simulink model "Encoder_X4"  (R2025a)
settings: Solver=FixedStepAuto  StartTime=0.0  StopTime=inf  FixedStep=0.001  RelTol=1e-3  EnableMultiTasking=on
libraries: stm32f4xxblockslib x5, stm32g4xxblockslib x2, simulink x1
settings Model: STM32="{\"EncoderBlockForG4\":[{\"ID\":\"untitled:1\"},{\"ID\":\"Lab3_Encoder:1\"},{\"ID\":\"Encoder:1\"},{\"ID\":\"Encoder_1:1\"},{\"ID\":\"Encoder_X4:147\"},{\"ID\":\"Encoder_X4:1\"},{\"ID\":\"Encoder_X1:147\"},{\"ID\":\"Encoder_X1:1\"},{\"ID\":\"Encoder_X2:147\"},{\"ID\":\"Encoder_X2:1\"}],\"DigitalPortRead\":[{\"ID\":\"Encoder:46\"},{\"ID\":\"Encoder:50\"},{\"ID\":\"Encoder:56\"},{\"ID\":\"Encoder_1:56\"},{\"ID\":\"Encoder_1:50\"},{\"ID\":\"Encoder_1:46\"},{\"ID\":\"Encoder_X4:56\"},{\"ID\":\"Encoder_X4:50\"},{\"ID\":\"Encoder_X4:46\"},{\"ID\":\"Encoder_X4:157\"},{\"ID\":\"Encoder_X4:158\"},{\"ID\":\"Encoder_X1:158\"},{\"ID\":\"Encoder_X1:157\"},{\"ID\":\"Encoder_X1:56\"},{\"ID\":\"Encoder_X1:50\"},{\"ID\":\"Encoder_X1:46\"},{\"ID\":\"Encoder_X2:158\"},{\"ID\":\"Encoder_X2:157\"},{\"ID\":\"Encoder_X2:50\"},{\"ID\":\"Encoder_X2:46\"}]}"  Creator=User  LastModifiedBy=rajap
settings OptimizationCC: DefaultParameterBehavior=Inlined  EnhancedBackFolding=on  PassReuseOutputArgsAs=Individual arguments  ZeroExternalMemoryAtStartup=off  ZeroInternalMemoryAtStartup=off  MaxStackSize=512  OptimizeBlockOrder=speed  DifferentSizesBufferReuse=on  OptimizationCustomize=off  EfficientTunableParamExpr=on
settings DebuggingCC: ParameterTunabilityLossMsg=error
settings HardwareCC: ProdBitPerPointer=32.0  ProdBitPerSizeT=32.0  ProdBitPerPtrDiffT=32.0  ProdLargestAtomicInteger=Long  ProdLargestAtomicFloat=Double  ProdWordSize=32.0  ProdLongLongMode=on  ProdHWDeviceType=ARM Compatible->ARM Cortex-M
settings SFSimCC: MATLABDynamicMemAlloc=off
settings RTWCC: SystemTargetFile=ert.tlc  HardwareBoard=STM32G4xx Based  TemplateMakefile=ert_default_tmf  Toolchain=GNU Tools for ARM Embedded Processors  Description=Embedded Coder
settings CodeAppCC: ForceParamTrailComments=on  IgnoreCustomStorageClasses=off  OperatorAnnotations=on  SimulinkDataObjDesc=on  SFDataObjDesc=on  InsertBlockDesc=on
settings ERTTargetCC: ExtModeTransport=3.0  ExtModeStaticAllocSize=2048.0  TargetLangStandard=C99 (ISO)  CodeReplacementLibrary=ARM Cortex-M  SupportContinuousTime=on

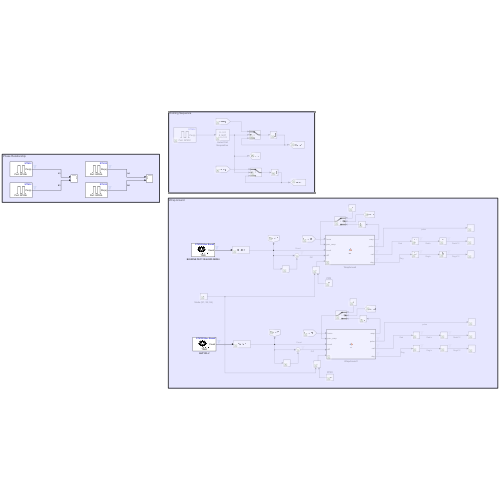
[thumbnail: Simulink's stored preview of the top-level diagram]
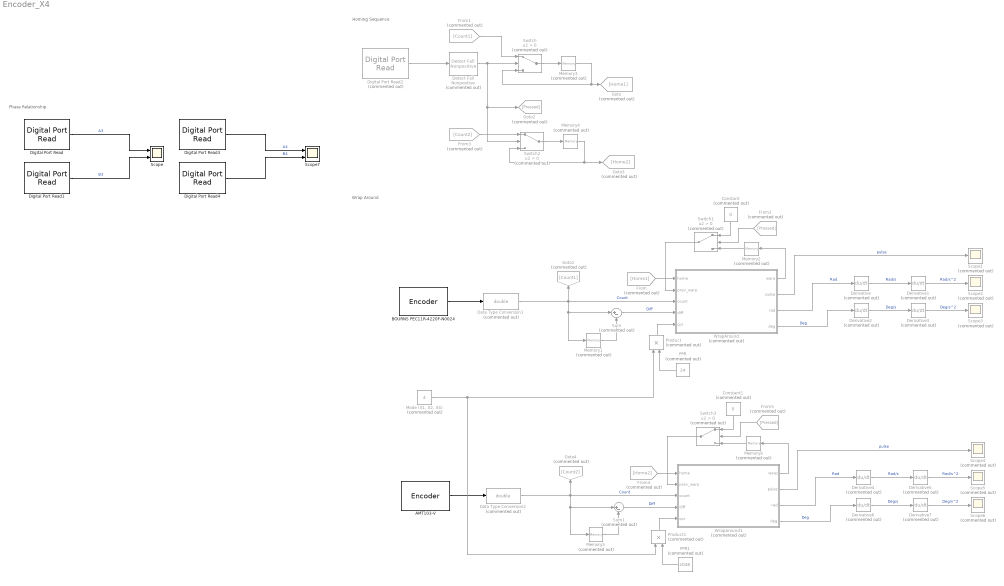
== system Encoder_X4 ==
  note: Wrap Around
  note: Homing Sequence
  note: Phase Relationship
  AMT103-V : stm32g4xxblockslib/Encoder  TimerModule=TIM4  EnableResetInput=off  OutputCountAfterFirstIndex=off  OutputValidIndex=off  OutputDirection=off  OutputStatus=off  SampleTime=-1
  BOURNS PEC11R-4220F-N0024 : stm32g4xxblockslib/Encoder  TimerModule=TIM3  EnableResetInput=off  OutputCountAfterFirstIndex=off  OutputValidIndex=off  OutputDirection=off  OutputStatus=off  SampleTime=-1
  Constant : Constant  Commented=on  Value=0
  Constant1 : Constant  Commented=on  Value=0
  Data Type Conversion1 : DataTypeConversion  Commented=on  OutDataTypeStr=double  SaturateOnIntegerOverflow=off  RndMeth=Floor
  Data Type Conversion2 : DataTypeConversion  Commented=on  OutDataTypeStr=double  SaturateOnIntegerOverflow=off  RndMeth=Floor
  Derivative{,1..7} (8 alike) : Derivative  Commented=on
  "Detect Fall Nonpositive " : simulink/Logic and Bit Operations/Detect Fall Nonpositive  Commented=on  vinit=0  OutDataTypeStr=boolean
  Digital Port Read : stm32f4xxblockslib/Digital Port Read  PortName=GPIOA  PinNumber=[6]  ReadOperation=on  IOAsArray=on  SampleTime=-1  EnableSimPort=off  hoistedMaskSrc=ECSoC/ECSimCodegen/Digital Port Read
  Digital Port Read1 : stm32f4xxblockslib/Digital Port Read  PortName=GPIOA  PinNumber=[4]  ReadOperation=on  IOAsArray=on  SampleTime=-1  EnableSimPort=off  hoistedMaskSrc=ECSoC/ECSimCodegen/Digital Port Read
  Digital Port Read2 : stm32f4xxblockslib/Digital Port Read  Commented=on  PortName=GPIOC  PinNumber=[13]  ReadOperation=on  IOAsArray=on  SampleTime=-1  EnableSimPort=off  hoistedMaskSrc=ECSoC/ECSimCodegen/Digital Port Read
  Digital Port Read3 : stm32f4xxblockslib/Digital Port Read  PortName=GPIOA  PinNumber=[11]  ReadOperation=on  IOAsArray=on  SampleTime=-1  EnableSimPort=off  hoistedMaskSrc=ECSoC/ECSimCodegen/Digital Port Read
  Digital Port Read4 : stm32f4xxblockslib/Digital Port Read  PortName=GPIOA  PinNumber=[12]  ReadOperation=on  IOAsArray=on  SampleTime=-1  EnableSimPort=off  hoistedMaskSrc=ECSoC/ECSimCodegen/Digital Port Read
  From : From  Commented=on  GotoTag=Home1
  From1 : From  Commented=on  GotoTag=Count1
  From2 : From  Commented=on  GotoTag=Pressed
  From3 : From  Commented=on  GotoTag=Count2
  From4 : From  Commented=on  GotoTag=Home2
  From5 : From  Commented=on  GotoTag=Pressed
  Goto : Goto  Commented=on  GotoTag=Home1
  Goto1 : Goto  Commented=on  GotoTag=Count1
  Goto2 : Goto  Commented=on  GotoTag=Pressed
  Goto3 : Goto  Commented=on  GotoTag=Home2
  Goto4 : Goto  Commented=on  GotoTag=Count2
  Memory{1..6} (6 alike) : Memory  Commented=on
  "Mode (X1, X2, X4)" : Constant  Commented=on  Value=4
  PPR : Constant  Commented=on  Value=24
  PPR1 : Constant  Commented=on  Value=2048
  Product : Product  Commented=on
  Product1 : Product  Commented=on
  Scope : Scope  NumInputPorts=2
  Scope{1..6} (6 alike) : Scope  Commented=on
      Scope2 settings: DataLoggingVariableName=ScopeData2
      Scope3 settings: DataLoggingVariableName=ScopeData3
      Scope4 settings: DataLoggingVariableName=ScopeData4
      Scope5 settings: DataLoggingVariableName=ScopeData5
      Scope6 settings: DataLoggingVariableName=ScopeData6
  Scope7 : Scope  NumInputPorts=2
      settings: DataLoggingVariableName=ScopeData7
  Sum : Sum  Commented=on  Inputs=|+-
  Sum1 : Sum  Commented=on  Inputs=|+-
  Switch{,1..3} (4 alike) : Switch  Commented=on  Criteria=u2 > Threshold  SaturateOnIntegerOverflow=off  InputSameDT=off
  WrapAround : MATLAB Function  Commented=on  TreatAsAtomicUnit=on
  WrapAround1 : MATLAB Function  Commented=on  TreatAsAtomicUnit=on
  wires:
  BOURNS PEC11R-4220F-N0024/1 -> Data Type Conversion1/1
  Data Type Conversion1/1 -> WrapAround/3(count), Goto1/1, Memory1/1, Sum/1  "Count"
  Derivative/1 -> Derivative1/1  "Rad/s"
  WrapAround/3(rad) -> Derivative/1  "Rad"
  WrapAround/4(deg) -> Derivative2/1  "Deg"
  Derivative2/1 -> Derivative3/1  "Deg/s"
  Derivative1/1 -> Scope2/1  "Rad/s^2"
  Derivative3/1 -> Scope3/1  "Deg/s^2"
  PPR/1 -> Product/2
  WrapAround/1(warp) -> Memory2/1
  Sum/1 -> WrapAround/4(diff)  "Diff"
  Memory1/1 -> Sum/2
  WrapAround/2(pulse) -> Scope1/1  "pulse"
  Product/1 -> WrapAround/5(cpr)
  Switch/1 -> Memory3/1
  Digital Port Read/1 -> Scope/1  "A3"
  Digital Port Read1/1 -> Scope/2  "B3"
  Digital Port Read2/1 -> "Detect Fall Nonpositive "/1
  Memory3/1 -> Switch/3, Goto/1
  "Detect Fall Nonpositive "/1 -> Goto2/1, Switch2/2, Switch/2
  Memory2/1 -> Switch1/3
  Constant/1 -> Switch1/1
  Switch1/1 -> WrapAround/2(prev_warp)
  From/1 -> WrapAround/1(home)
  From1/1 -> Switch/1
  From2/1 -> Switch1/2
  From3/1 -> Switch2/1
  Memory4/1 -> Switch2/3, Goto3/1
  Switch2/1 -> Memory4/1
  From4/1 -> WrapAround1/1(home)
  Derivative4/1 -> Derivative5/1  "Rad/s"
  Sum1/1 -> WrapAround1/4(diff)  "Diff"
  Data Type Conversion2/1 -> WrapAround1/3(count), Goto4/1, Sum1/1, Memory5/1  "Count"
  WrapAround1/3(rad) -> Derivative4/1  "Rad"
  AMT103-V/1 -> Data Type Conversion2/1
  Derivative6/1 -> Derivative7/1  "Deg/s"
  Switch3/1 -> WrapAround1/2(prev_warp)
  WrapAround1/1(warp) -> Memory6/1
  Constant1/1 -> Switch3/1
  Memory6/1 -> Switch3/3
  WrapAround1/4(deg) -> Derivative6/1  "Deg"
  Derivative5/1 -> Scope5/1  "Rad/s^2"
  WrapAround1/2(pulse) -> Scope4/1  "pulse"
  Derivative7/1 -> Scope6/1  "Deg/s^2"
  From5/1 -> Switch3/2
  "Mode (X1, X2, X4)"/1 -> Product1/1, Product/1
  PPR1/1 -> Product1/2
  Memory5/1 -> Sum1/2
  Product1/1 -> WrapAround1/5(cpr)
  Digital Port Read4/1 -> Scope7/2  "B4"
  Digital Port Read3/1 -> Scope7/1  "A4"

== matlab function Encoder_X4/WrapAround1 ==
  data: warp output; home input; prev_warp input; pulse output; count input; diff input; cpr input; rad output; deg output
function [warp, pulse, rad, deg]= fcn(home, prev_warp, count, diff, cpr)

if diff <= -cpr * 0.5
    warp = prev_warp + 1;
    pulse = count + (warp * cpr);
elseif diff >= cpr * 0.5
    warp = prev_warp - 1;
    pulse = count - (warp * cpr);
else
    warp = prev_warp;
    pulse = count + (warp * cpr);
end

pulse = pulse - home;
rad = (pulse * 2 * pi) / cpr;
deg = rad2deg(rad);

== matlab function Encoder_X4/WrapAround ==
  data: warp output; home input; prev_warp input; pulse output; count input; diff input; cpr input; rad output; deg output
function [warp, pulse, rad, deg]= fcn(home, prev_warp, count, diff, cpr)

if diff <= -cpr * 0.5
    warp = prev_warp + 1;
    pulse = count + (warp * cpr);
elseif diff >= cpr * 0.5
    warp = prev_warp - 1;
    pulse = count - (warp * cpr);
else
    warp = prev_warp;
    pulse = count + (warp * cpr);
end

pulse = pulse - home;
rad = (pulse * 2 * pi) / cpr;
deg = rad2deg(rad);
